simulink model "g"  (R2024b)
settings: Solver=FixedStepAuto  StartTime=0.0  StopTime=25  FixedStep=0.01  RelTol=1e-3
libraries: simulink x1
settings Model: Creator=john  LastModifiedBy=john

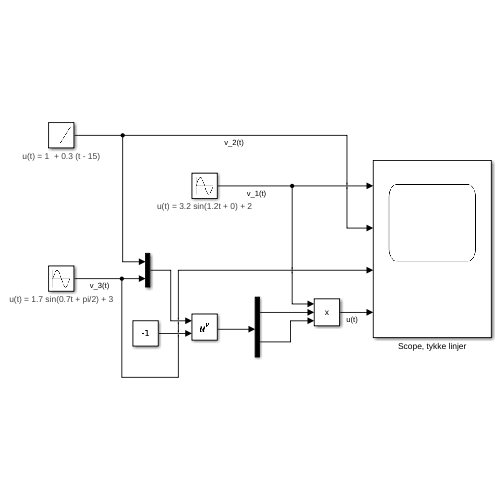
[thumbnail: Simulink's stored preview of the top-level diagram]
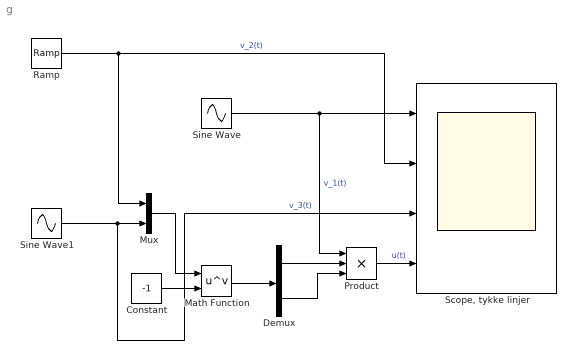
== system g ==
  Constant : Constant  Value=-1
  Demux : Demux  Outputs=2
  Math Function : Math  Operator=pow
  Mux : Mux  Inputs=2
  Product : Product  Inputs=3
  Ramp : simulink/Sources/Ramp  slope=0.3  start=15  InitialOutput=1
      settings: AttributesFormatString="u(t) = %<InitialOutput>  + %<slope> (t - %<start>)"
  "Scope, tykke linjer" : Scope  NumInputPorts=4
  Sine Wave : Sin  Amplitude=3.2  Bias=2  Frequency=1.2  SampleTime=0
      settings: AttributesFormatString=u(t) = %<Amplitude> sin(%<Frequency>t + %<Phase>) + %<Bias>
  Sine Wave1 : Sin  Amplitude=1.7  Bias=3  Frequency=0.7  Phase=pi/2  SampleTime=0
      settings: AttributesFormatString=u(t) = %<Amplitude> sin(%<Frequency>t + %<Phase>) + %<Bias>
  wires:
  Product/1 -> "Scope, tykke linjer"/4  "u(t)"
  Math Function/1 -> Demux/1
  Demux/2 -> Product/3
  Constant/1 -> Math Function/2
  Demux/1 -> Product/2
  Sine Wave/1 -> "Scope, tykke linjer"/1, Product/1  "v_1(t)"
  Mux/1 -> Math Function/1
  Sine Wave1/1 -> "Scope, tykke linjer"/3, Mux/2  "v_3(t)"
  Ramp/1 -> Mux/1, "Scope, tykke linjer"/2  "v_2(t)"
